simulink model "rlHumanMuscleModel"  (R2023b)
settings: Solver=VariableStepAuto  StartTime=0.0  StopTime=inf  RelTol=1e-3
model workspace (MATLAB code in the model file):
  | mCart = 1;
  | mPend = 1;
  | g = 9.81;
  | L = 0.5;
  | theta0 = 180;
  | Kd = 10;
undefined symbols (not defined in the file): ankle_r_MEE, ankle_r_MEF, board_freq, foot, hip_r_MEE, hip_r_MEF, knee_r_MEE, knee_r_MEF, lower_leg, Param_ankle_MEE, Param_ankle_MEF, Param_hip_MEE, Param_hip_MEF, Param_knee_MEE, Param_knee_MEF, u_cutoff, upper_body, upper_leg, X, Y, Z
libraries: sm_lib x22, nesl_utility x19, Library_mtu_simulink x12, rllib x1
settings Model: Creator=The MathWorks, Inc.  LastModifiedBy=r
settings SolverCC: AlgebraicLoopSolver=TrustRegion
settings DataIOCC: TimeSaveName=T  SignalLoggingName=LoggedSigs
settings DebuggingCC: UnconnectedInputMsg=warning  UnconnectedOutputMsg=warning  UnconnectedLineMsg=warning  ArithmeticOperatorsInVariantConditions=warning
settings ModelReferenceCC: EnableRefExpFcnMdlSchedulingChecks=on
settings SFSimCC: CustomCodeUndefinedFunction=UseInterfaceOnly
settings ExplorerConfigSet: InternalSimMechanicsExplorerSettings="<ExplorerConfiguration><canonicalview>default</canonicalview><AnimationSetting><BasePlaybackSpeed>1.0</BasePlaybackSpeed><PlaybackSpeedFactor>1.0</PlaybackSpeedFactor></AnimationSetting><TilePanel><TileInfo><Tiles Columns=\"1\" Count=\"1\" Rows=\"1\"><Column Weight=\"1\"/><Row Weight=\"1\"/><Tile Height=\"1\" Width=\"1\" X=\"0\" Y=\"0\"/></Tiles></TileInfo><SceneInfo><SceneViewer><BGColor><R>0.60000002384185791</R><G>0.60000002384185791</G><B>0.60000002384185791</B></BGColor><Camera><DoPerspective>off</DoPerspective><Position><X>0</X><Y>0.883749991655349731</Y><Z>1.40844246480054913</Z></Position><Center><X>0</X><Y>0.883749991655349731</Y><Z>0</Z></Center><Up><X>0</X><Y>1</Y><Z>-0</Z></Up><ViewLimDist>1</ViewLimDist><YLim>0.915412517189979624</YLim><XLim>1.33857490721176275</XLim></Camera></SceneViewer></SceneInfo></TilePanel><MechEditorPanel><Cameras/><GfxPanelCameraMap/><VideoCreator><PlaybackSpeedRatio>1.0</PlaybackSpeedRatio><FrameRate>30</FrameRate><VideoFormat>Motion JPEG AVI</VideoFormat><FrameSize>auto</FrameSize></VideoCreator></MechEditorPanel></ExplorerConfiguration>"

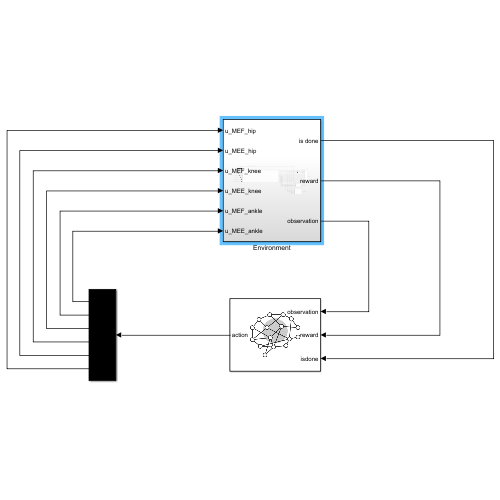
[thumbnail: Simulink's stored preview of the top-level diagram]
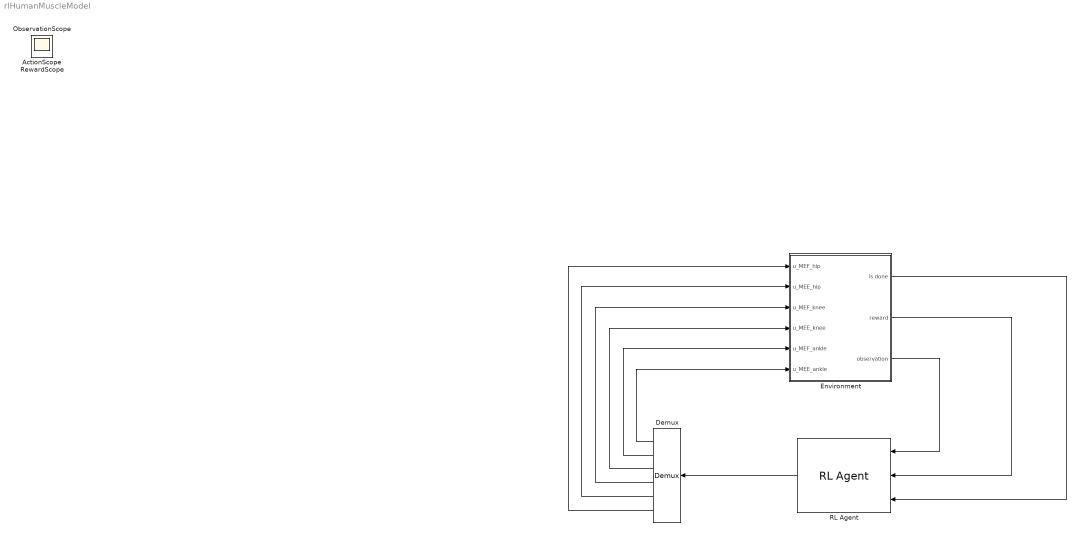
== system rlHumanMuscleModel ==
  Demux : Demux  Outputs=6
  Environment : Subsystem
  RL Agent : rllib/RL Agent  Agent=agent  ExternalActionAsInput=off  ProvideLastAction=off  ProvideCumRwd=off  TreatAsDirectFeedthrough=on  UseStrictObservationDataTypes=off
  ActionScope : Scope
  ObservationScope : Scope
  RewardScope : Scope
  wires:
  Environment/1(is done) -> RL Agent/3
  Environment/2(reward) -> RL Agent/2
  Environment/3(observation) -> RL Agent/1
  Demux/1 -> Environment/6(u_MEE_ankle)
  Demux/2 -> Environment/5(u_MEF_ankle)
  Demux/3 -> Environment/4(u_MEE_knee)
  Demux/4 -> Environment/3(u_MEF_knee)
  Demux/5 -> Environment/2(u_MEE_hip)
  Demux/6 -> Environment/1(u_MEF_hip)
  RL Agent/1 -> Demux/1

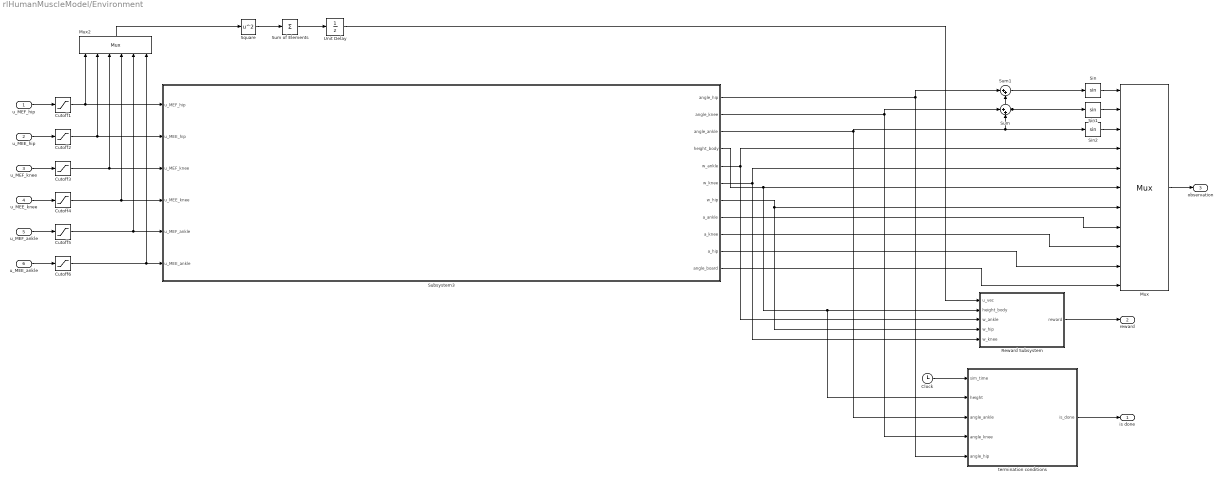
== system rlHumanMuscleModel/Environment ==
  u_MEF_hip : Inport
  u_MEE_hip : Inport  Port=2
  u_MEF_knee : Inport  Port=3
  u_MEE_knee : Inport  Port=4
  u_MEF_ankle : Inport  Port=5
  u_MEE_ankle : Inport  Port=6
  Clock : Clock
  Cutoff{1..6} (6 alike) : Saturate  UpperLimit=u_cutoff  LowerLimit=0
  Mux : Mux  Inputs=11
  Mux2 : Mux  Inputs=6
  Reward Subsystem : Subsystem
  Sin : Trigonometry
  Sin1 : Trigonometry
  Sin2 : Trigonometry
  Square : Math  Operator=square
  Subsystem3 : Subsystem
  Sum : Sum  Inputs=|++
  Sum of Elements : Sum  Inputs=+
  Sum1 : Sum  Inputs=|++
  Unit Delay : UnitDelay  SampleTime=-1  HasFrameUpgradeWarning=on
  "termination conditions " : MATLAB Function  TreatAsAtomicUnit=on
  is done : Outport  VectorParamsAs1DForOutWhenUnconnected=off
  reward : Outport  Port=2  VectorParamsAs1DForOutWhenUnconnected=off
  observation : Outport  Port=3
  wires:
  u_MEE_hip/1 -> Cutoff2/1
  u_MEF_hip/1 -> Cutoff1/1
  Cutoff1/1 -> Mux2/1, Subsystem3/1(u_MEF_hip)
  Cutoff2/1 -> Mux2/2, Subsystem3/2(u_MEE_hip)
  Cutoff3/1 -> Mux2/3, Subsystem3/3(u_MEF_knee)
  u_MEF_knee/1 -> Cutoff3/1
  u_MEE_knee/1 -> Cutoff4/1
  Cutoff4/1 -> Subsystem3/4(u_MEE_knee), Mux2/4
  Cutoff5/1 -> Subsystem3/5(u_MEF_ankle), Mux2/5
  u_MEF_ankle/1 -> Cutoff5/1
  Cutoff6/1 -> Mux2/6, Subsystem3/6(u_MEE_ankle)
  u_MEE_ankle/1 -> Cutoff6/1
  Mux/1 -> observation/1
  Subsystem3/6(w_knee) -> Reward Subsystem/5(w_knee), Mux/5
  Subsystem3/5(w_ankle) -> Reward Subsystem/3(w_ankle), Mux/4
  Subsystem3/4(height_body) -> Mux/6, "termination conditions "/2(height), Reward Subsystem/2(height_body)
  Reward Subsystem/1(reward) -> reward/1
  Subsystem3/7(w_hip) -> Reward Subsystem/4(w_hip), Mux/7
  Unit Delay/1 -> Reward Subsystem/1(u_vec)
  Mux2/1 -> Square/1
  Square/1 -> Sum of Elements/1
  Sum of Elements/1 -> Unit Delay/1
  Sin/1 -> Mux/1
  Sin1/1 -> Mux/2
  Sin2/1 -> Mux/3
  Sum/1 -> Sum1/2, Sin1/1
  Sum1/1 -> Sin/1
  Subsystem3/1(angle_hip) -> "termination conditions "/5(angle_hip), Sum1/1
  "termination conditions "/1(is_done) -> is done/1
  Clock/1 -> "termination conditions "/1(sim_time)
  Subsystem3/3(angle_ankle) -> "termination conditions "/3(angle_ankle), Sum/2, Sin2/1
  Subsystem3/2(angle_knee) -> "termination conditions "/4(angle_knee), Sum/1
  Subsystem3/8(a_ankle) -> Mux/8
  Subsystem3/9(a_knee) -> Mux/9
  Subsystem3/10(a_hip) -> Mux/10
  Subsystem3/11(angle_board) -> Mux/11

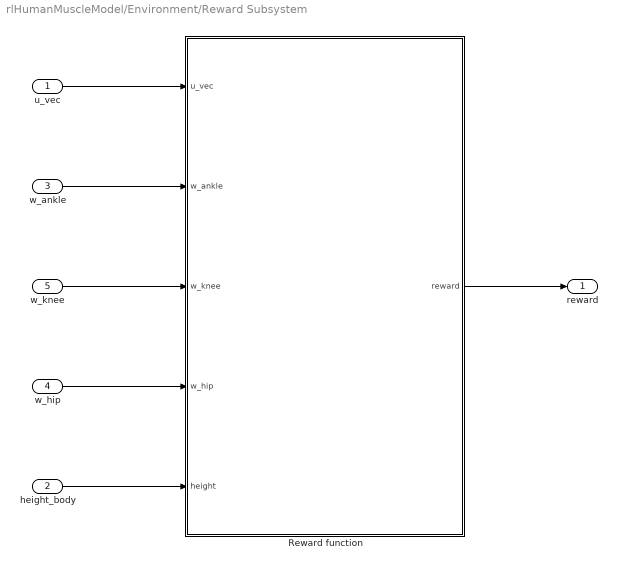
== system rlHumanMuscleModel/Environment/Reward Subsystem ==
  u_vec : Inport
  height_body : Inport  Port=2
  w_ankle : Inport  Port=3
  w_hip : Inport  Port=4
  w_knee : Inport  Port=5
  Reward function : MATLAB Function  TreatAsAtomicUnit=on
  reward : Outport
  wires:
  Reward function/1(reward) -> reward/1
  w_knee/1 -> Reward function/3(w_knee)
  w_ankle/1 -> Reward function/2(w_ankle)
  w_hip/1 -> Reward function/4(w_hip)
  height_body/1 -> Reward function/5(height)
  u_vec/1 -> Reward function/1(u_vec)

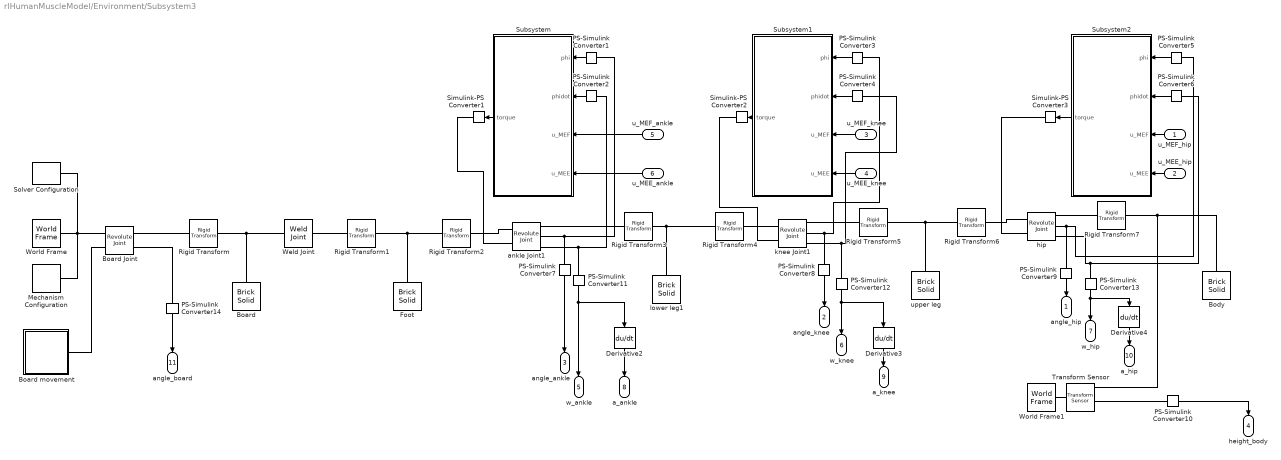
== system rlHumanMuscleModel/Environment/Subsystem3 ==
  u_MEF_hip : Inport
  u_MEE_hip : Inport  Port=2
  u_MEF_knee : Inport  Port=3
  u_MEE_knee : Inport  Port=4
  u_MEF_ankle : Inport  Port=5
  u_MEE_ankle : Inport  Port=6
  Board : sm_lib/Body Elements/Brick Solid  GraphicAmbientColor=[0.15 0.15 0.15 1.0]  BasedOnType=Density  BrickDimensions=[2.0 0.01 0.01]  BrickDimensionsUnits=m  CenterOfMass=[0 0 0]  CenterOfMassUnits=m  GraphicDiffuseColor=[0.5 0.5 0.5]  Density=1000  DensityUnits=kg/m^3  DoExposeReferenceFrame=on  GraphicEmissiveColor=[0.0 0.0 0.0 1.0]  ExportEntireGeometry=off  SerializedFrames=<Frames/>  MarkerShape=Sphere  MarkerSize=10  GraphicType=FromGeometry  InertiaType=Custom  Mass=300  MassUnits=kg  MomentsOfInertia=[0 0 0.24]  MomentsOfInertiaUnits=kg*m^2  GraphicOpacity=1.0  ProductsOfInertia=[0 0 0]  ProductsOfInertiaUnits=kg*m^2  GraphicShininess=75  GraphicSpecularColor=[0.5 0.5 0.5 1.0]  GraphicVisPropType=SimpleVisualProperties
  Board Joint : sm_lib/Joints/Revolute Joint  JointMode=Normal  SenseConstraintForce=off  SenseConstraintForceX=off  SenseConstraintForceY=off  SenseConstraintForceZ=off  SenseConstraintTorque=off  SenseConstraintTorqueX=off  SenseConstraintTorqueY=off  SenseConstraintTorqueZ=off  SenseTotalForce=off  SenseTotalForceX=off  SenseTotalForceY=off  SenseTotalForceZ=off  SenseTotalTorque=off  SenseTotalTorqueX=off  SenseTotalTorqueY=off  SenseTotalTorqueZ=off  CompositeWrenchDir=FollowerOnBase  CompositeWrenchFrame=BaseFrame  EquilibriumPosition=0  EquilibriumPositionUnits=deg  SpringStiffness=0  SpringStiffnessUnits=N*m/deg  DampingCoefficient=0  DampingCoefficientUnits=N*m/(deg/s)  TorqueActuationMode=ComputedTorque  MotionActuationMode=InputMotion  SensePosition=on  SenseVelocity=off  SenseAcceleration=off  SenseTorqueForce=off  SenseLowerLimitTorqueForce=off  SenseUpperLimitTorqueForce=off  LowerLimitSpecify=off  LowerLimitBound=-10  LowerLimitBoundUnits=deg  LowerLimitStiffness=1000  LowerLimitStiffnessUnits=N*m/rad  LowerLimitDamping=10  LowerLimitDampingUnits=N*m*s/rad  LowerLimitTransitionRegionWidth=0.1  LowerLimitTransitionRegionWidthUnits=deg  UpperLimitSpecify=off  UpperLimitBound=10  UpperLimitBoundUnits=deg  UpperLimitStiffness=1000  UpperLimitStiffnessUnits=N*m/rad  UpperLimitDamping=10  UpperLimitDampingUnits=N*m*s/rad  UpperLimitTransitionRegionWidth=0.1  UpperLimitTransitionRegionWidthUnits=deg  PositionTargetSpecify=off  PositionTargetPriority=High  PositionTargetValue=0.35  PositionTargetValueUnits=rad  VelocityTargetSpecify=off  VelocityTargetPriority=High  VelocityTargetValue=0  VelocityTargetValueUnits=deg/s
  Board movement : Subsystem
  Body : sm_lib/Body Elements/Brick Solid  GraphicAmbientColor=[0.15 0.15 0.15 1.0]  BasedOnType=Density  BrickDimensions=[0.01 upper_body.length 0.01]  BrickDimensionsUnits=m  CenterOfMass=[0 -upper_body.com 0]  CenterOfMassUnits=m  GraphicDiffuseColor=[0.2 0.2 1.0]  Density=1000  DensityUnits=kg/m^3  DoExposeReferenceFrame=on  GraphicEmissiveColor=[0.0 0.0 0.0 1.0]  ExportEntireGeometry=off  SerializedFrames=<Frames/>  MarkerShape=Sphere  MarkerSize=10  GraphicType=FromGeometry  InertiaType=Custom  Mass=upper_body.mass  MassUnits=kg  MomentsOfInertia=[0 0 upper_body.inertia]  MomentsOfInertiaUnits=kg*m^2  GraphicOpacity=1.0  ProductsOfInertia=[0 0 0]  ProductsOfInertiaUnits=kg*m^2  GraphicShininess=75  GraphicSpecularColor=[0.5 0.5 0.5 1.0]  GraphicVisPropType=SimpleVisualProperties
  Derivative2 : Derivative
  Derivative3 : Derivative
  Derivative4 : Derivative
  Foot : sm_lib/Body Elements/Brick Solid  GraphicAmbientColor=[0.15 0.15 0.15 1.0]  BasedOnType=Density  BrickDimensions=[foot.length 0.01 0.01]  BrickDimensionsUnits=m  CenterOfMass=[0 foot.com 0]  CenterOfMassUnits=m  GraphicDiffuseColor=[1.0 0.2 0.0]  Density=1000  DensityUnits=kg/m^3  DoExposeReferenceFrame=on  GraphicEmissiveColor=[0.0 0.0 0.0 1.0]  ExportEntireGeometry=off  SerializedFrames=<Frames/>  MarkerShape=Sphere  MarkerSize=10  GraphicType=FromGeometry  InertiaType=Custom  Mass=foot.mass  MassUnits=kg  MomentsOfInertia=[0 0 foot.inertia]  MomentsOfInertiaUnits=kg*m^2  GraphicOpacity=1.0  ProductsOfInertia=[0 0 0]  ProductsOfInertiaUnits=kg*m^2  GraphicShininess=75  GraphicSpecularColor=[0.5 0.5 0.5 1.0]  GraphicVisPropType=SimpleVisualProperties
  Mechanism Configuration : sm_lib/Utilities/Mechanism Configuration  UniformGravity=Constant  GravityVector="[0  -9.80665 0]"  GravityVectorUnits=m/s^2  LinearizationDelta=0.001  JointModeTransitionNonlinearIterations=2
  PS-Simulink Converter{1..14} (14 alike) : nesl_utility/PS-Simulink Converter  PhysicalDomain=network_engine_domain  SubClassName=ps_output  LeftPortType=input  RightPortType=output  PseudoPeriodic=off  Frequencies=[]  VectorFormat=inherit  Unit=inherit  AffineConversion=off
  Rigid Transform : sm_lib/Frames and Transforms/Rigid Transform  TranslationMethod=StandardAxis  TranslationStandardOffset=0  TranslationStandardOffsetUnits=m  TranslationStandardAxis=+Y  TranslationCartesianOffset=[0 0 0]  TranslationCartesianOffsetUnits=m  TranslationROffset=0  TranslationROffsetUnits=m  TranslationZOffset=0  TranslationZOffsetUnits=m  TranslationThetaOffset=0  TranslationThetaOffsetUnits=deg  RotationMethod=None  RotationAngleUnits=deg  RotationStandardAxis=+Z  RotationAngle=0.0  RotationArbitraryAxis=[0 0 1]  FollAlignAxisA=+X  BaseAlignAxisA=+Y  FollAlignAxisB=+Y  BaseAlignAxisB=+Z  RotationSequenceAxes=FollowerAxes  RotationSequence=XYX  RotationSequenceAngles=[0 0 0]  RotationSequenceAnglesUnits=deg  RotationMatrix=[1 0 0; 0 1 0; 0 0 1]  Quaternion=[1 0 0 0]
  Rigid Transform1 : sm_lib/Frames and Transforms/Rigid Transform  TranslationMethod=StandardAxis  TranslationStandardOffset=0.01  TranslationStandardOffsetUnits=m  TranslationStandardAxis=+Y  TranslationCartesianOffset=[0 0 0]  TranslationCartesianOffsetUnits=m  TranslationROffset=0  TranslationROffsetUnits=m  TranslationZOffset=0  TranslationZOffsetUnits=m  TranslationThetaOffset=0  TranslationThetaOffsetUnits=deg  RotationMethod=None  RotationAngleUnits=deg  RotationStandardAxis=+Z  RotationAngle=0.0  RotationArbitraryAxis=[0 0 1]  FollAlignAxisA=+X  BaseAlignAxisA=+Y  FollAlignAxisB=+Y  BaseAlignAxisB=+Z  RotationSequenceAxes=FollowerAxes  RotationSequence=XYX  RotationSequenceAngles=[0 0 0]  RotationSequenceAnglesUnits=deg  RotationMatrix=[1 0 0; 0 1 0; 0 0 1]  Quaternion=[1 0 0 0]
  Rigid Transform2 : sm_lib/Frames and Transforms/Rigid Transform  TranslationMethod=StandardAxis  TranslationStandardOffset=foot.length/2  TranslationStandardOffsetUnits=m  TranslationStandardAxis=+X  TranslationCartesianOffset=[0 0 0]  TranslationCartesianOffsetUnits=m  TranslationROffset=0  TranslationROffsetUnits=m  TranslationZOffset=0  TranslationZOffsetUnits=m  TranslationThetaOffset=0  TranslationThetaOffsetUnits=deg  RotationMethod=None  RotationAngleUnits=deg  RotationStandardAxis=+Z  RotationAngle=0.0  RotationArbitraryAxis=[0 0 1]  FollAlignAxisA=+X  BaseAlignAxisA=+Y  FollAlignAxisB=+Y  BaseAlignAxisB=+Z  RotationSequenceAxes=FollowerAxes  RotationSequence=XYX  RotationSequenceAngles=[0 0 0]  RotationSequenceAnglesUnits=deg  RotationMatrix=[1 0 0; 0 1 0; 0 0 1]  Quaternion=[1 0 0 0]
  Rigid Transform3 : sm_lib/Frames and Transforms/Rigid Transform  TranslationMethod=StandardAxis  TranslationStandardOffset=lower_leg.length/2  TranslationStandardOffsetUnits=m  TranslationStandardAxis=+Y  TranslationCartesianOffset=[0 0 0]  TranslationCartesianOffsetUnits=m  TranslationROffset=0  TranslationROffsetUnits=m  TranslationZOffset=0  TranslationZOffsetUnits=m  TranslationThetaOffset=0  TranslationThetaOffsetUnits=deg  RotationMethod=None  RotationAngleUnits=deg  RotationStandardAxis=+Z  RotationAngle=0.0  RotationArbitraryAxis=[0 0 1]  FollAlignAxisA=+X  BaseAlignAxisA=+Y  FollAlignAxisB=+Y  BaseAlignAxisB=+Z  RotationSequenceAxes=FollowerAxes  RotationSequence=XYX  RotationSequenceAngles=[0 0 0]  RotationSequenceAnglesUnits=deg  RotationMatrix=[1 0 0; 0 1 0; 0 0 1]  Quaternion=[1 0 0 0]
  Rigid Transform4 : sm_lib/Frames and Transforms/Rigid Transform  TranslationMethod=StandardAxis  TranslationStandardOffset=lower_leg.length/2  TranslationStandardOffsetUnits=m  TranslationStandardAxis=+Y  TranslationCartesianOffset=[0 0 0]  TranslationCartesianOffsetUnits=m  TranslationROffset=0  TranslationROffsetUnits=m  TranslationZOffset=0  TranslationZOffsetUnits=m  TranslationThetaOffset=0  TranslationThetaOffsetUnits=deg  RotationMethod=None  RotationAngleUnits=deg  RotationStandardAxis=+Z  RotationAngle=0.0  RotationArbitraryAxis=[0 0 1]  FollAlignAxisA=+X  BaseAlignAxisA=+Y  FollAlignAxisB=+Y  BaseAlignAxisB=+Z  RotationSequenceAxes=FollowerAxes  RotationSequence=XYX  RotationSequenceAngles=[0 0 0]  RotationSequenceAnglesUnits=deg  RotationMatrix=[1 0 0; 0 1 0; 0 0 1]  Quaternion=[1 0 0 0]
  Rigid Transform5 : sm_lib/Frames and Transforms/Rigid Transform  TranslationMethod=StandardAxis  TranslationStandardOffset=upper_leg.length/2  TranslationStandardOffsetUnits=m  TranslationStandardAxis=+Y  TranslationCartesianOffset=[0 0 0]  TranslationCartesianOffsetUnits=m  TranslationROffset=0  TranslationROffsetUnits=m  TranslationZOffset=0  TranslationZOffsetUnits=m  TranslationThetaOffset=0  TranslationThetaOffsetUnits=deg  RotationMethod=None  RotationAngleUnits=deg  RotationStandardAxis=+Z  RotationAngle=0.0  RotationArbitraryAxis=[0 0 1]  FollAlignAxisA=+X  BaseAlignAxisA=+Y  FollAlignAxisB=+Y  BaseAlignAxisB=+Z  RotationSequenceAxes=FollowerAxes  RotationSequence=XYX  RotationSequenceAngles=[0 0 0]  RotationSequenceAnglesUnits=deg  RotationMatrix=[1 0 0; 0 1 0; 0 0 1]  Quaternion=[1 0 0 0]
  Rigid Transform6 : sm_lib/Frames and Transforms/Rigid Transform  TranslationMethod=StandardAxis  TranslationStandardOffset=upper_leg.length/2  TranslationStandardOffsetUnits=m  TranslationStandardAxis=+Y  TranslationCartesianOffset=[0 0 0]  TranslationCartesianOffsetUnits=m  TranslationROffset=0  TranslationROffsetUnits=m  TranslationZOffset=0  TranslationZOffsetUnits=m  TranslationThetaOffset=0  TranslationThetaOffsetUnits=deg  RotationMethod=None  RotationAngleUnits=deg  RotationStandardAxis=+Z  RotationAngle=0.0  RotationArbitraryAxis=[0 0 1]  FollAlignAxisA=+X  BaseAlignAxisA=+Y  FollAlignAxisB=+Y  BaseAlignAxisB=+Z  RotationSequenceAxes=FollowerAxes  RotationSequence=XYX  RotationSequenceAngles=[0 0 0]  RotationSequenceAnglesUnits=deg  RotationMatrix=[1 0 0; 0 1 0; 0 0 1]  Quaternion=[1 0 0 0]
  Rigid Transform7 : sm_lib/Frames and Transforms/Rigid Transform  TranslationMethod=StandardAxis  TranslationStandardOffset=upper_body.length/2  TranslationStandardOffsetUnits=m  TranslationStandardAxis=+Y  TranslationCartesianOffset=[0 0 0]  TranslationCartesianOffsetUnits=m  TranslationROffset=0  TranslationROffsetUnits=m  TranslationZOffset=0  TranslationZOffsetUnits=m  TranslationThetaOffset=0  TranslationThetaOffsetUnits=deg  RotationMethod=None  RotationAngleUnits=deg  RotationStandardAxis=+Z  RotationAngle=0.0  RotationArbitraryAxis=[0 0 1]  FollAlignAxisA=+X  BaseAlignAxisA=+Y  FollAlignAxisB=+Y  BaseAlignAxisB=+Z  RotationSequenceAxes=FollowerAxes  RotationSequence=XYX  RotationSequenceAngles=[0 0 0]  RotationSequenceAnglesUnits=deg  RotationMatrix=[1 0 0; 0 1 0; 0 0 1]  Quaternion=[1 0 0 0]
  Simulink-PS Converter1 : nesl_utility/Simulink-PS Converter  PhysicalDomain=network_engine_domain  SubClassName=ps_input  LeftPortType=input  RightPortType=output  PseudoPeriodic=off  Frequencies=[]  NoiseDistribution=none  NoiseParameters=[]  Unit=1  AffineConversion=off  FilteringAndDerivatives=provide  SimscapeFilterOrder=1  InputFilterTimeConstant=0.001  UdotUserProvided=0
  Simulink-PS Converter2 : nesl_utility/Simulink-PS Converter  PhysicalDomain=network_engine_domain  SubClassName=ps_input  LeftPortType=input  RightPortType=output  PseudoPeriodic=off  Frequencies=[]  NoiseDistribution=none  NoiseParameters=[]  Unit=1  AffineConversion=off  FilteringAndDerivatives=provide  SimscapeFilterOrder=1  InputFilterTimeConstant=0.001  UdotUserProvided=0
  Simulink-PS Converter3 : nesl_utility/Simulink-PS Converter  PhysicalDomain=network_engine_domain  SubClassName=ps_input  LeftPortType=input  RightPortType=output  PseudoPeriodic=off  Frequencies=[]  NoiseDistribution=none  NoiseParameters=[]  Unit=1  AffineConversion=off  FilteringAndDerivatives=provide  SimscapeFilterOrder=1  InputFilterTimeConstant=0.001  UdotUserProvided=0
  Solver Configuration : nesl_utility/Solver Configuration  PhysicalDomain=network_engine_domain  SubClassName=solver  LeftPortType=input  RightPortType=generic  Tones=[]  Harmonics=[]  SimulateNoise=off  Profile=off  UseLocalSampling=off  EnableSwitchedLinearOptims=on  FrequencyDomain=off  UseCCode=off  RelTol=0.001  AbsTol=1e-06  MinStep=1e-09  ToWorkspace=off  RevertToSquareIcSolve=off  NumHomotopyIterations=100  PhasorMode=off  PhasorModeNumHarmonics=1  ConsistencySolver=NEWTON_XTOL_AFTER_FTOL  IndexReductionMethod=DerivativeReplacement  DoDC=off  ResidualTolerance=1e-09  ConsistencyTolSource=GLOBAL  ConsistencyAbsTol=0.001  ConsistencyRelTol=0.001  ConsistencyTolFactor=0.001  UseLocalSolver=off  LocalSolverChoice=NE_BACKWARD_EULER_ADVANCER  ResolveIndetEquations=on  FunctionEvalNumThread=1  LocalSolverSampleTime=0.001  DoFixedCost=off  MaxNonlinIter=3  MaxModeIter=2  ComputeImpulses=off  ImpulseIterations=2  LinearAlgebra=Sparse  LinearAlgebraNumThread=0  EquationFormulation=NE_TIME_EF  DelaysMemoryBudget=1024  AutomaticFiltering=on  FilteringTimeConstant=0.001  PartitionStorageMethod=AS_NEEDED  PartitionMemoryBudget=1024  PartitionMethod=FAST  MultibodyUseLocalSolver=off  MultibodyLocalSolverChoice=ODE1  MultibodyLocalSolverSampleTime=0.001
  Subsystem : Subsystem
  Subsystem1 : Subsystem
  Subsystem2 : Subsystem
  Transform Sensor : sm_lib/Frames and Transforms/Transform Sensor  MeasurementFrame=World  RotationSequence=XYX  SenseAngle=off  SenseAxis=off  SenseQ=off  SenseR=off  SenseRotationSequence=off  SenseOmegaX=off  SenseOmegaY=off  SenseOmegaZ=off  SenseOmega=off  SenseQDot=off  SenseRDot=off  SenseRotationSequenceDot=off  SenseAlphaX=off  SenseAlphaY=off  SenseAlphaZ=off  SenseAlpha=off  SenseQDDot=off  SenseRDDot=off  SenseX=on  SenseY=on  SenseZ=on  SenseXYZ=off  SenseRad=off  SenseAzim=off  SenseDist=off  SenseInc=off  SenseXDot=off  SenseYDot=off  SenseZDot=off  SenseXYZDot=off  SenseRadDot=off  SenseAzimDot=off  SenseDistDot=off  SenseIncDot=off  SenseXDDot=off  SenseYDDot=off  SenseZDDot=off  SenseXYZDDot=off  SenseRadDDot=off  SenseAzimDDot=off  SenseDistDDot=off  SenseIncDDot=off
  Weld Joint : sm_lib/Joints/Weld Joint  JointMode=Normal  SenseConstraintForce=off  SenseConstraintForceX=off  SenseConstraintForceY=off  SenseConstraintForceZ=off  SenseConstraintTorque=off  SenseConstraintTorqueX=off  SenseConstraintTorqueY=off  SenseConstraintTorqueZ=off  SenseTotalForce=off  SenseTotalForceX=off  SenseTotalForceY=off  SenseTotalForceZ=off  SenseTotalTorque=off  SenseTotalTorqueX=off  SenseTotalTorqueY=off  SenseTotalTorqueZ=off  CompositeWrenchDir=FollowerOnBase  CompositeWrenchFrame=BaseFrame
  World Frame : sm_lib/Frames and Transforms/World Frame
  World Frame1 : sm_lib/Frames and Transforms/World Frame
  ankle Joint1 : sm_lib/Joints/Revolute Joint  JointMode=Normal  SenseConstraintForce=off  SenseConstraintForceX=off  SenseConstraintForceY=off  SenseConstraintForceZ=off  SenseConstraintTorque=off  SenseConstraintTorqueX=off  SenseConstraintTorqueY=off  SenseConstraintTorqueZ=off  SenseTotalForce=off  SenseTotalForceX=off  SenseTotalForceY=off  SenseTotalForceZ=off  SenseTotalTorque=off  SenseTotalTorqueX=off  SenseTotalTorqueY=off  SenseTotalTorqueZ=off  CompositeWrenchDir=FollowerOnBase  CompositeWrenchFrame=BaseFrame  EquilibriumPosition=0  EquilibriumPositionUnits=deg  SpringStiffness=0  SpringStiffnessUnits=N*m/deg  DampingCoefficient=0  DampingCoefficientUnits=N*m/(deg/s)  TorqueActuationMode=InputTorque  MotionActuationMode=ComputedMotion  SensePosition=on  SenseVelocity=on  SenseAcceleration=off  SenseTorqueForce=off  SenseLowerLimitTorqueForce=off  SenseUpperLimitTorqueForce=off  LowerLimitSpecify=on  LowerLimitBound=angle_ankle_min  LowerLimitBoundUnits=deg  LowerLimitStiffness=1000  LowerLimitStiffnessUnits=N*m/rad  LowerLimitDamping=10  LowerLimitDampingUnits=N*m*s/rad  LowerLimitTransitionRegionWidth=0.1  LowerLimitTransitionRegionWidthUnits=deg  UpperLimitSpecify=on  UpperLimitBound=angle_ankle_max  UpperLimitBoundUnits=deg  UpperLimitStiffness=1000  UpperLimitStiffnessUnits=N*m/rad  UpperLimitDamping=10  UpperLimitDampingUnits=N*m*s/rad  UpperLimitTransitionRegionWidth=0.1  UpperLimitTransitionRegionWidthUnits=deg  PositionTargetSpecify=off  PositionTargetPriority=High  PositionTargetValue=0.35  PositionTargetValueUnits=rad  VelocityTargetSpecify=off  VelocityTargetPriority=High  VelocityTargetValue=0  VelocityTargetValueUnits=deg/s
  hip : sm_lib/Joints/Revolute Joint  JointMode=Normal  SenseConstraintForce=off  SenseConstraintForceX=off  SenseConstraintForceY=off  SenseConstraintForceZ=off  SenseConstraintTorque=off  SenseConstraintTorqueX=off  SenseConstraintTorqueY=off  SenseConstraintTorqueZ=off  SenseTotalForce=off  SenseTotalForceX=off  SenseTotalForceY=off  SenseTotalForceZ=off  SenseTotalTorque=off  SenseTotalTorqueX=off  SenseTotalTorqueY=off  SenseTotalTorqueZ=off  CompositeWrenchDir=FollowerOnBase  CompositeWrenchFrame=BaseFrame  EquilibriumPosition=0  EquilibriumPositionUnits=deg  SpringStiffness=0  SpringStiffnessUnits=N*m/deg  DampingCoefficient=0  DampingCoefficientUnits=N*m/(deg/s)  TorqueActuationMode=InputTorque  MotionActuationMode=ComputedMotion  SensePosition=on  SenseVelocity=on  SenseAcceleration=off  SenseTorqueForce=off  SenseLowerLimitTorqueForce=off  SenseUpperLimitTorqueForce=off  LowerLimitSpecify=on  LowerLimitBound=angle_hip_min  LowerLimitBoundUnits=deg  LowerLimitStiffness=1000  LowerLimitStiffnessUnits=N*m/rad  LowerLimitDamping=10  LowerLimitDampingUnits=N*m*s/rad  LowerLimitTransitionRegionWidth=0.1  LowerLimitTransitionRegionWidthUnits=deg  UpperLimitSpecify=on  UpperLimitBound=angle_hip_max  UpperLimitBoundUnits=deg  UpperLimitStiffness=1000  UpperLimitStiffnessUnits=N*m/rad  UpperLimitDamping=10  UpperLimitDampingUnits=N*m*s/rad  UpperLimitTransitionRegionWidth=0.1  UpperLimitTransitionRegionWidthUnits=deg  PositionTargetSpecify=off  PositionTargetPriority=High  PositionTargetValue=0  PositionTargetValueUnits=deg  VelocityTargetSpecify=off  VelocityTargetPriority=High  VelocityTargetValue=0  VelocityTargetValueUnits=deg/s
  knee Joint1 : sm_lib/Joints/Revolute Joint  JointMode=Normal  SenseConstraintForce=off  SenseConstraintForceX=off  SenseConstraintForceY=off  SenseConstraintForceZ=off  SenseConstraintTorque=off  SenseConstraintTorqueX=off  SenseConstraintTorqueY=off  SenseConstraintTorqueZ=off  SenseTotalForce=off  SenseTotalForceX=off  SenseTotalForceY=off  SenseTotalForceZ=off  SenseTotalTorque=off  SenseTotalTorqueX=off  SenseTotalTorqueY=off  SenseTotalTorqueZ=off  CompositeWrenchDir=FollowerOnBase  CompositeWrenchFrame=BaseFrame  EquilibriumPosition=0  EquilibriumPositionUnits=deg  SpringStiffness=0  SpringStiffnessUnits=N*m/deg  DampingCoefficient=0  DampingCoefficientUnits=N*m/(deg/s)  TorqueActuationMode=InputTorque  MotionActuationMode=ComputedMotion  SensePosition=on  SenseVelocity=on  SenseAcceleration=off  SenseTorqueForce=off  SenseLowerLimitTorqueForce=off  SenseUpperLimitTorqueForce=off  LowerLimitSpecify=on  LowerLimitBound=angle_knee_min  LowerLimitBoundUnits=deg  LowerLimitStiffness=1000  LowerLimitStiffnessUnits=N*m/rad  LowerLimitDamping=10  LowerLimitDampingUnits=N*m*s/rad  LowerLimitTransitionRegionWidth=0.1  LowerLimitTransitionRegionWidthUnits=deg  UpperLimitSpecify=on  UpperLimitBound=angle_knee_max  UpperLimitBoundUnits=deg  UpperLimitStiffness=1000  UpperLimitStiffnessUnits=N*m/rad  UpperLimitDamping=10  UpperLimitDampingUnits=N*m*s/rad  UpperLimitTransitionRegionWidth=0.1  UpperLimitTransitionRegionWidthUnits=deg  PositionTargetSpecify=off  PositionTargetPriority=High  PositionTargetValue=0  PositionTargetValueUnits=deg  VelocityTargetSpecify=off  VelocityTargetPriority=High  VelocityTargetValue=0  VelocityTargetValueUnits=deg/s
  lower leg1 : sm_lib/Body Elements/Brick Solid  GraphicAmbientColor=[0.15 0.15 0.15 1.0]  BasedOnType=Density  BrickDimensions=[0.01 lower_leg.length 0.01]  BrickDimensionsUnits=m  CenterOfMass=[0 lower_leg.com 0]  CenterOfMassUnits=m  GraphicDiffuseColor=[0.5 0.5 0.5]  Density=1000  DensityUnits=kg/m^3  DoExposeReferenceFrame=on  GraphicEmissiveColor=[0.0 0.0 0.0 1.0]  ExportEntireGeometry=off  SerializedFrames=<Frames/>  MarkerShape=Sphere  MarkerSize=10  GraphicType=FromGeometry  InertiaType=Custom  Mass=lower_leg.mass  MassUnits=kg  MomentsOfInertia=[0 0 lower_leg.inertia]  MomentsOfInertiaUnits=kg*m^2  GraphicOpacity=1.0  ProductsOfInertia=[0 0 0]  ProductsOfInertiaUnits=kg*m^2  GraphicShininess=75  GraphicSpecularColor=[0.5 0.5 0.5 1.0]  GraphicVisPropType=SimpleVisualProperties
  upper leg : sm_lib/Body Elements/Brick Solid  GraphicAmbientColor=[0.15 0.15 0.15 1.0]  BasedOnType=Density  BrickDimensions=[0.01 upper_leg.length 0.01]  BrickDimensionsUnits=m  CenterOfMass=[0 upper_leg.com 0]  CenterOfMassUnits=m  GraphicDiffuseColor=[0.2 0.2 1.0]  Density=1000  DensityUnits=kg/m^3  DoExposeReferenceFrame=on  GraphicEmissiveColor=[0.0 0.0 0.0 1.0]  ExportEntireGeometry=off  SerializedFrames=<Frames/>  MarkerShape=Sphere  MarkerSize=10  GraphicType=FromGeometry  InertiaType=Custom  Mass=upper_leg.mass  MassUnits=kg  MomentsOfInertia=[0 0 upper_leg.inertia]  MomentsOfInertiaUnits=kg*m^2  GraphicOpacity=1.0  ProductsOfInertia=[0 0 0]  ProductsOfInertiaUnits=kg*m^2  GraphicShininess=75  GraphicSpecularColor=[0.5 0.5 0.5 1.0]  GraphicVisPropType=SimpleVisualProperties
  angle_hip : Outport
  angle_knee : Outport  Port=2
  angle_ankle : Outport  Port=3
  height_body : Outport  Port=4
  w_ankle : Outport  Port=5
  w_knee : Outport  Port=6
  w_hip : Outport  Port=7
  a_ankle : Outport  Port=8
  a_knee : Outport  Port=9
  a_hip : Outport  Port=10
  angle_board : Outport  Port=11
  wires:
  u_MEE_knee/1 -> Subsystem1/4(u_MEE)
  u_MEE_ankle/1 -> Subsystem/4(u_MEE)
  PS-Simulink Converter1/1 -> Subsystem/1(phi)
  Subsystem/1(torque) -> Simulink-PS Converter1/1
  PS-Simulink Converter6/1 -> Subsystem2/2(phidot)
  u_MEF_hip/1 -> Subsystem2/3(u_MEF)
  PS-Simulink Converter2/1 -> Subsystem/2(phidot)
  PS-Simulink Converter3/1 -> Subsystem1/1(phi)
  PS-Simulink Converter5/1 -> Subsystem2/1(phi)
  Subsystem1/1(torque) -> Simulink-PS Converter2/1
  Subsystem2/1(torque) -> Simulink-PS Converter3/1
  PS-Simulink Converter4/1 -> Subsystem1/2(phidot)
  u_MEE_hip/1 -> Subsystem2/4(u_MEE)
  u_MEF_ankle/1 -> Subsystem/3(u_MEF)
  u_MEF_knee/1 -> Subsystem1/3(u_MEF)
  PS-Simulink Converter7/1 -> angle_ankle/1
  PS-Simulink Converter8/1 -> angle_knee/1
  PS-Simulink Converter9/1 -> angle_hip/1
  PS-Simulink Converter10/1 -> height_body/1
  PS-Simulink Converter11/1 -> Derivative2/1, w_ankle/1
  Derivative2/1 -> a_ankle/1
  Derivative3/1 -> a_knee/1
  PS-Simulink Converter12/1 -> Derivative3/1, w_knee/1
  Derivative4/1 -> a_hip/1
  PS-Simulink Converter13/1 -> Derivative4/1, w_hip/1
  PS-Simulink Converter14/1 -> angle_board/1
  connections:
  ankle Joint1/RConn2 -- PS-Simulink Converter1/LConn1 -- PS-Simulink Converter7/LConn1
  Rigid Transform7/LConn1 -- hip/RConn1
  Simulink-PS Converter2/RConn1 -- knee Joint1/LConn2
  PS-Simulink Converter5/LConn1 -- hip/RConn2 -- PS-Simulink Converter9/LConn1
  hip/RConn3 -- PS-Simulink Converter6/LConn1 -- PS-Simulink Converter13/LConn1
  Simulink-PS Converter3/RConn1 -- hip/LConn2
  upper leg/RConn1 -- Rigid Transform5/RConn1 -- Rigid Transform6/LConn1
  Rigid Transform2/RConn1 -- ankle Joint1/LConn1
  Rigid Transform6/RConn1 -- hip/LConn1
  ankle Joint1/RConn3 -- PS-Simulink Converter2/LConn1 -- PS-Simulink Converter11/LConn1
  Board Joint/RConn1 -- Rigid Transform/LConn1
  Body/RConn1 -- Rigid Transform7/RConn1 -- Transform Sensor/RConn1
  Rigid Transform3/LConn1 -- ankle Joint1/RConn1
  PS-Simulink Converter3/LConn1 -- knee Joint1/RConn2 -- PS-Simulink Converter8/LConn1
  knee Joint1/RConn1 -- Rigid Transform5/LConn1
  Simulink-PS Converter1/RConn1 -- ankle Joint1/LConn2
  knee Joint1/RConn3 -- PS-Simulink Converter12/LConn1 -- PS-Simulink Converter4/LConn1
  knee Joint1/LConn1 -- Rigid Transform4/RConn1
  lower leg1/RConn1 -- Rigid Transform3/RConn1 -- Rigid Transform4/LConn1
  Rigid Transform1/LConn1 -- Weld Joint/RConn1
  Foot/RConn1 -- Rigid Transform2/LConn1 -- Rigid Transform1/RConn1
  Mechanism Configuration/RConn1 -- Solver Configuration/RConn1 -- Board Joint/LConn1 -- World Frame/RConn1
  Board/RConn1 -- Weld Joint/LConn1 -- Rigid Transform/RConn1
  World Frame1/RConn1 -- Transform Sensor/LConn1
  PS-Simulink Converter10/LConn1 -- Transform Sensor/RConn3
  Board Joint/RConn2 -- PS-Simulink Converter14/LConn1
  Board movement/RConn1 -- Board Joint/LConn2

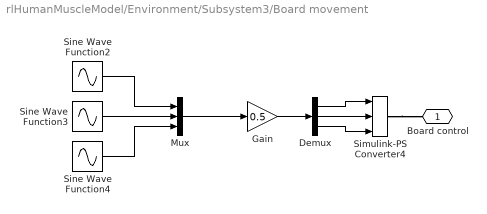
== system rlHumanMuscleModel/Environment/Subsystem3/Board movement ==
  Demux : Demux  Outputs=3
  Gain : Gain  Gain=0.5
  Mux : Mux  Inputs=3
  Simulink-PS Converter4 : nesl_utility/Simulink-PS Converter  PhysicalDomain=network_engine_domain  SubClassName=ps_input  LeftPortType=input  RightPortType=output  PseudoPeriodic=off  Frequencies=[]  NoiseDistribution=none  NoiseParameters=[]  Unit=1  AffineConversion=off  FilteringAndDerivatives=provide  SimscapeFilterOrder=1  InputFilterTimeConstant=0.001  UdotUserProvided=2
  Sine Wave Function2 : Sin  Amplitude=0.5  Frequency=board_freq  SampleTime=0
  Sine Wave Function3 : Sin  Amplitude=0.5*board_freq  Frequency=board_freq  Phase=pi/2  SampleTime=0
  Sine Wave Function4 : Sin  Amplitude=-0.5*board_freq*board_freq  Frequency=board_freq  SampleTime=0
  Board control : PMIOPort  Side=Right
  wires:
  Sine Wave Function3/1 -> Mux/2
  Sine Wave Function4/1 -> Mux/3
  Sine Wave Function2/1 -> Mux/1
  Gain/1 -> Demux/1
  Demux/3 -> Simulink-PS Converter4/3
  Demux/1 -> Simulink-PS Converter4/1
  Demux/2 -> Simulink-PS Converter4/2
  Mux/1 -> Gain/1
  connections:
  Simulink-PS Converter4/RConn1 -- Board control/RConn1

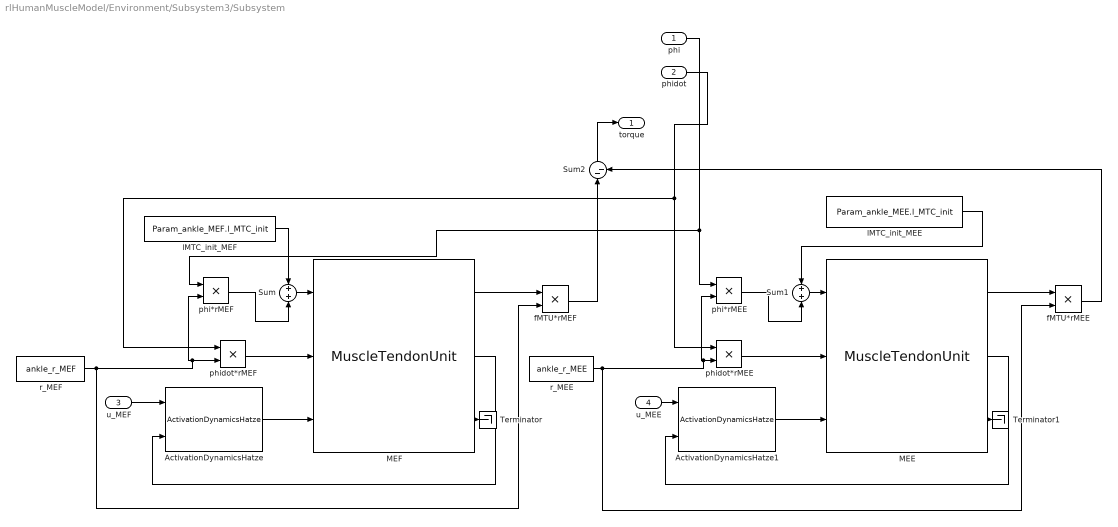
== system rlHumanMuscleModel/Environment/Subsystem3/Subsystem ==
  phi : Inport
  phidot : Inport  Port=2
  u_MEF : Inport  Port=3
  u_MEE : Inport  Port=4
  ActivationDynamicsHatze : Library_mtu_simulink/ActivationDynamicsHatze  Act_Param=Param_ankle_MEF.ActDyn  Mus_Param=Param_ankle_MEF
  ActivationDynamicsHatze1 : Library_mtu_simulink/ActivationDynamicsHatze  Act_Param=Param_ankle_MEE.ActDyn  Mus_Param=Param_ankle_MEE
  MEE : Library_mtu_simulink/MuscleTendonUnit  Mus_Param=Param_ankle_MEE
  MEF : Library_mtu_simulink/MuscleTendonUnit  Mus_Param=Param_ankle_MEF
  Sum : Sum  Inputs=+|+
  Sum1 : Sum  Inputs=+|+
  Sum2 : Sum  Inputs=|--
  Terminator : Terminator
  Terminator1 : Terminator
  fMTU*rMEE : Product
  fMTU*rMEF : Product
  lMTC_init_MEE : Constant  Value=Param_ankle_MEE.l_MTC_init
  lMTC_init_MEF : Constant  Value=Param_ankle_MEF.l_MTC_init
  phi*rMEE : Product
  phi*rMEF : Product
  phidot*rMEE : Product
  phidot*rMEF : Product
  r_MEE : Constant  Value=ankle_r_MEE
  r_MEF : Constant  Value=ankle_r_MEF
  torque : Outport
  wires:
  phi/1 -> phi*rMEE/1, phi*rMEF/1
  lMTC_init_MEF/1 -> Sum/1
  phidot*rMEF/1 -> MEF/2
  r_MEF/1 -> fMTU*rMEF/2, phi*rMEF/2, phidot*rMEF/2
  fMTU*rMEE/1 -> Sum2/2
  MEF/2 -> ActivationDynamicsHatze/2
  lMTC_init_MEE/1 -> Sum1/1
  ActivationDynamicsHatze/1 -> MEF/3
  phi*rMEE/1 -> Sum1/2
  Sum1/1 -> MEE/1
  MEF/3 -> Terminator/1
  phi*rMEF/1 -> Sum/2
  MEE/2 -> ActivationDynamicsHatze1/2
  r_MEE/1 -> fMTU*rMEE/2, phi*rMEE/2, phidot*rMEE/2
  MEE/1 -> fMTU*rMEE/1
  Sum/1 -> MEF/1
  MEE/3 -> Terminator1/1
  phidot/1 -> phidot*rMEE/1, phidot*rMEF/1
  phidot*rMEE/1 -> MEE/2
  MEF/1 -> fMTU*rMEF/1
  fMTU*rMEF/1 -> Sum2/1
  ActivationDynamicsHatze1/1 -> MEE/3
  Sum2/1 -> torque/1
  u_MEF/1 -> ActivationDynamicsHatze/1
  u_MEE/1 -> ActivationDynamicsHatze1/1

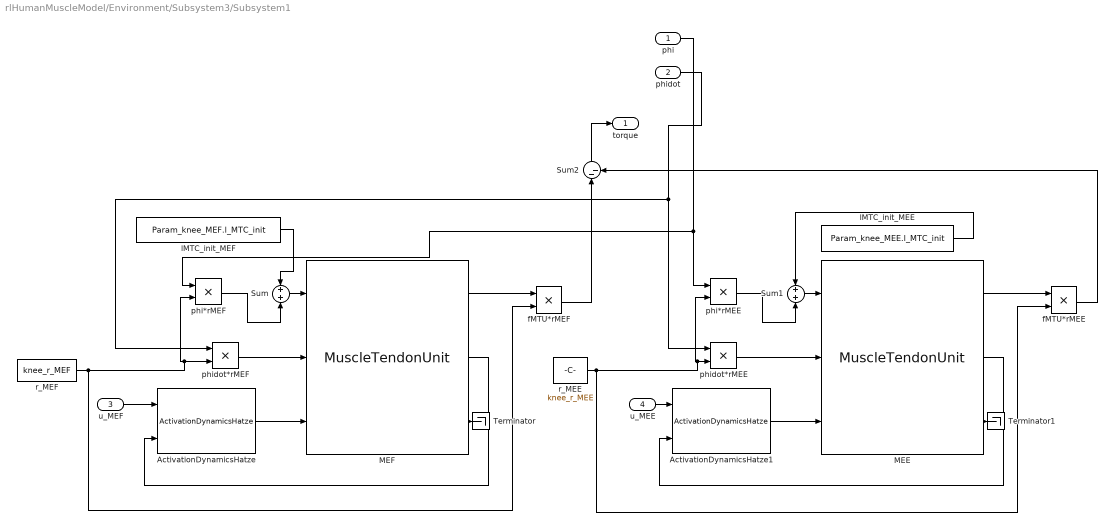
== system rlHumanMuscleModel/Environment/Subsystem3/Subsystem1 ==
  phi : Inport
  phidot : Inport  Port=2
  u_MEF : Inport  Port=3
  u_MEE : Inport  Port=4
  ActivationDynamicsHatze : Library_mtu_simulink/ActivationDynamicsHatze  Act_Param=Param_knee_MEF.ActDyn  Mus_Param=Param_knee_MEF
  ActivationDynamicsHatze1 : Library_mtu_simulink/ActivationDynamicsHatze  Act_Param=Param_knee_MEE.ActDyn  Mus_Param=Param_knee_MEE
  MEE : Library_mtu_simulink/MuscleTendonUnit  Mus_Param=Param_knee_MEE
  MEF : Library_mtu_simulink/MuscleTendonUnit  Mus_Param=Param_knee_MEF
  Sum : Sum  Inputs=+|+
  Sum1 : Sum  Inputs=+|+
  Sum2 : Sum  Inputs=|--
  Terminator : Terminator
  Terminator1 : Terminator
  fMTU*rMEE : Product
  fMTU*rMEF : Product
  lMTC_init_MEE : Constant  Value=Param_knee_MEE.l_MTC_init
  lMTC_init_MEF : Constant  Value=Param_knee_MEF.l_MTC_init
  phi*rMEE : Product
  phi*rMEF : Product
  phidot*rMEE : Product
  phidot*rMEF : Product
  r_MEE : Constant  Value=knee_r_MEE
  r_MEF : Constant  Value=knee_r_MEF
  torque : Outport
  wires:
  phi/1 -> phi*rMEE/1, phi*rMEF/1
  lMTC_init_MEF/1 -> Sum/1
  phidot*rMEF/1 -> MEF/2
  r_MEF/1 -> fMTU*rMEF/2, phi*rMEF/2, phidot*rMEF/2
  fMTU*rMEE/1 -> Sum2/2
  MEF/2 -> ActivationDynamicsHatze/2
  lMTC_init_MEE/1 -> Sum1/1
  ActivationDynamicsHatze/1 -> MEF/3
  phi*rMEE/1 -> Sum1/2
  Sum1/1 -> MEE/1
  MEF/3 -> Terminator/1
  phi*rMEF/1 -> Sum/2
  MEE/2 -> ActivationDynamicsHatze1/2
  r_MEE/1 -> fMTU*rMEE/2, phi*rMEE/2, phidot*rMEE/2
  MEE/1 -> fMTU*rMEE/1
  Sum/1 -> MEF/1
  MEE/3 -> Terminator1/1
  phidot/1 -> phidot*rMEE/1, phidot*rMEF/1
  phidot*rMEE/1 -> MEE/2
  MEF/1 -> fMTU*rMEF/1
  fMTU*rMEF/1 -> Sum2/1
  ActivationDynamicsHatze1/1 -> MEE/3
  Sum2/1 -> torque/1
  u_MEF/1 -> ActivationDynamicsHatze/1
  u_MEE/1 -> ActivationDynamicsHatze1/1

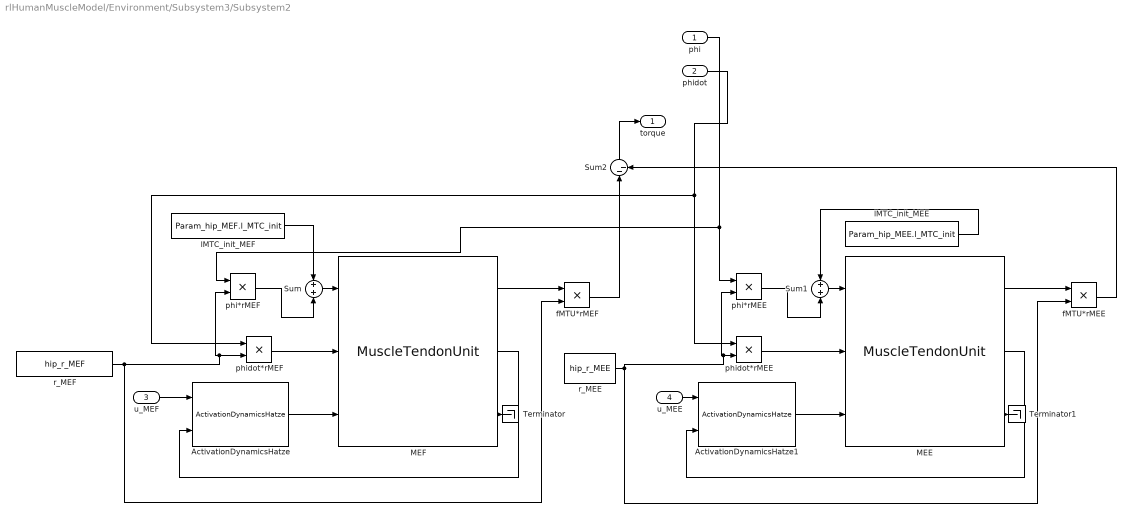
== system rlHumanMuscleModel/Environment/Subsystem3/Subsystem2 ==
  phi : Inport
  phidot : Inport  Port=2
  u_MEF : Inport  Port=3
  u_MEE : Inport  Port=4
  ActivationDynamicsHatze : Library_mtu_simulink/ActivationDynamicsHatze  Act_Param=Param_hip_MEF.ActDyn  Mus_Param=Param_hip_MEF
  ActivationDynamicsHatze1 : Library_mtu_simulink/ActivationDynamicsHatze  Act_Param=Param_hip_MEE.ActDyn  Mus_Param=Param_hip_MEE
  MEE : Library_mtu_simulink/MuscleTendonUnit  Mus_Param=Param_hip_MEE
  MEF : Library_mtu_simulink/MuscleTendonUnit  Mus_Param=Param_hip_MEF
  Sum : Sum  Inputs=+|+
  Sum1 : Sum  Inputs=+|+
  Sum2 : Sum  Inputs=|--
  Terminator : Terminator
  Terminator1 : Terminator
  fMTU*rMEE : Product
  fMTU*rMEF : Product
  lMTC_init_MEE : Constant  Value=Param_hip_MEE.l_MTC_init
  lMTC_init_MEF : Constant  Value=Param_hip_MEF.l_MTC_init
  phi*rMEE : Product
  phi*rMEF : Product
  phidot*rMEE : Product
  phidot*rMEF : Product
  r_MEE : Constant  Value=hip_r_MEE
  r_MEF : Constant  Value=hip_r_MEF
  torque : Outport
  wires:
  phi/1 -> phi*rMEE/1, phi*rMEF/1
  lMTC_init_MEF/1 -> Sum/1
  phidot*rMEF/1 -> MEF/2
  r_MEF/1 -> fMTU*rMEF/2, phi*rMEF/2, phidot*rMEF/2
  fMTU*rMEE/1 -> Sum2/2
  MEF/2 -> ActivationDynamicsHatze/2
  lMTC_init_MEE/1 -> Sum1/1
  ActivationDynamicsHatze/1 -> MEF/3
  phi*rMEE/1 -> Sum1/2
  Sum1/1 -> MEE/1
  MEF/3 -> Terminator/1
  phi*rMEF/1 -> Sum/2
  MEE/2 -> ActivationDynamicsHatze1/2
  r_MEE/1 -> phi*rMEE/2, phidot*rMEE/2, fMTU*rMEE/2
  MEE/1 -> fMTU*rMEE/1
  Sum/1 -> MEF/1
  MEE/3 -> Terminator1/1
  phidot/1 -> phidot*rMEE/1, phidot*rMEF/1
  phidot*rMEE/1 -> MEE/2
  MEF/1 -> fMTU*rMEF/1
  fMTU*rMEF/1 -> Sum2/1
  ActivationDynamicsHatze1/1 -> MEE/3
  Sum2/1 -> torque/1
  u_MEF/1 -> ActivationDynamicsHatze/1
  u_MEE/1 -> ActivationDynamicsHatze1/1

== matlab function rlHumanMuscleModel/Environment/termination conditions  ==
  data: sim_time input; height input; angle_ankle input; angle_knee input; angle_hip input; is_done output
function is_done = fcn(sim_time, height, angle_ankle, angle_knee, angle_hip)
    epsilon = 0.1;
    is_done = false;

    % angles in radians
    Tf = 20.0;
    angle_ankle_min = -50/180*pi;
    angle_ankle_max = 50/180*pi;
    angle_knee_min = -135/180*pi;
    angle_knee_max = 20/180*pi; 
    angle_hip_min = -40/180*pi;
    angle_hip_max = 110/180*pi;

    if sim_time > Tf
        is_done = true;
        return;
    end

    if height < 0
        is_done = true;
        return;
    end

    if angle_ankle < angle_ankle_min * (1 + epsilon)
        is_done = true;
        return;
    end
    if angle_knee < angle_knee_min * (1 + epsilon)
        is_done = true;
        return;
    end
    if angle_hip < angle_hip_min * (1 + epsilon)
        is_done = true;
        return;
    end

    if angle_ankle > angle_ankle_max * (1 + epsilon)
        is_done = true;
        return;
    end
    if angle_knee > angle_knee_max * (1 + epsilon)
        is_done = true;
        return;
    end
    if angle_hip > angle_hip_max * (1 + epsilon)
        is_done = true;
        return;
    end
end

== matlab function rlHumanMuscleModel/Environment/Reward Subsystem/Reward function ==
  data: u_vec input; reward output; w_ankle input; w_knee input; w_hip input; height input
function reward = fcn(u_vec, w_ankle, w_knee, w_hip, height)
    % height: 0.0 m to 1.3 m
    % u_sum: 0.0 to 1.0
    % w_ankle: -1.0 to 1.0
    % w_knee: -3.0 to 3.0
    % w_hip: -3.0 to 3.0
    
    height_reward = height^2;
    duration_reward = 1.0;
    regulation_reward = -0.1 * u_vec;
    speed_reward = -0.075*(w_ankle^2 + w_knee^2 + w_hip^2);
    reward = height_reward + duration_reward + regulation_reward + speed_reward;
end
